simulink model "linealizacion_"  (R2024a)
settings: Solver=VariableStepAuto  StartTime=0.0  StopTime=10.0  RelTol=1e-3
settings Model: Creator=alfre
settings RTWCC: GPUComputeCapability=3.5

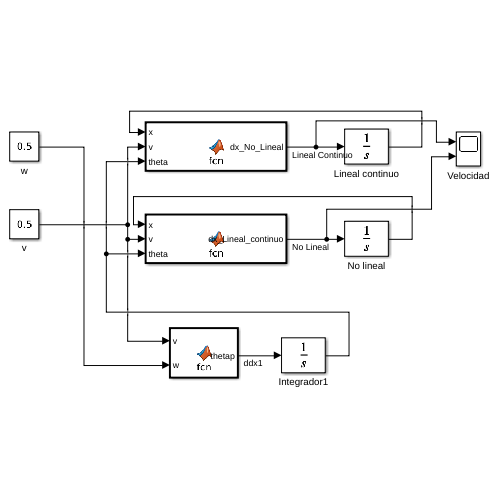
[thumbnail: Simulink's stored preview of the top-level diagram]
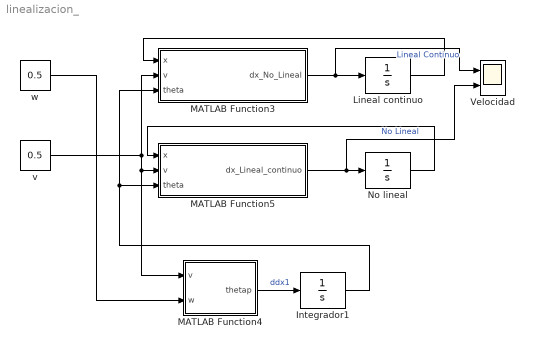
== system linealizacion_ ==
  Integrador1 : Integrator  ContinuousStateAttributes="\"dx\""
  Lineal continuo : Integrator  ContinuousStateAttributes="\"dx\""
  MATLAB Function3 : MATLAB Function  TreatAsAtomicUnit=on
  MATLAB Function4 : MATLAB Function  TreatAsAtomicUnit=on
  MATLAB Function5 : MATLAB Function  TreatAsAtomicUnit=on
  No lineal : Integrator  ContinuousStateAttributes="\"dx\""
  Velocidad : Scope  NumInputPorts=2
  v : Constant  Value=0.5
  w : Constant  Value=0.5
  wires:
  Lineal continuo/1 -> MATLAB Function3/1(x)
  Integrador1/1 -> MATLAB Function5/3(theta), MATLAB Function3/3(theta)
  MATLAB Function3/1(dx_No_Lineal) -> Velocidad/1, Lineal continuo/1  "Lineal Continuo"
  No lineal/1 -> MATLAB Function5/1(x)
  w/1 -> MATLAB Function4/2(w)
  MATLAB Function5/1(dx_Lineal_continuo) -> Velocidad/2, No lineal/1  "No Lineal"
  MATLAB Function4/1(thetap) -> Integrador1/1  "ddx1"
  v/1 -> MATLAB Function3/2(v), MATLAB Function5/2(v), MATLAB Function4/1(v)

== matlab function linealizacion_/MATLAB Function3 ==
  data: x input; v input; dx_No_Lineal output; theta input
function dx_No_Lineal = fcn(x, v, theta)
dx_No_Lineal= v*cos(theta);
dx_Lineal_continuo = -v*sin(theta)*theta
dx_Lineal_discreto = x -v*sin(theta)*theta

== matlab function linealizacion_/MATLAB Function4 ==
  data: v input; w input; thetap output
function thetap = fcn(v,w)
r=1;
w=v/r;
thetap=w;

== matlab function linealizacion_/MATLAB Function5 ==
  data: x input; v input; dx_Lineal_continuo output; theta input
function dx_Lineal_continuo = fcn(x, v, theta)
dx_No_Lineal= v*cos(theta);
dx_Lineal_continuo = -v*sin(theta)*theta
dx_Lineal_discreto = x -v*sin(theta)*theta
